simulink model "Ae483_project"  (R2018a)
settings: Solver=ode15s  StartTime=0.0  StopTime=50  RelTol=1e-4
values from neighbouring files (symbols this model uses):
  A_10_ang = [-1.3336 -0.5124 0.1399 ... (first row only)    [Ae483Project.m]
  A_10_ang_ob = bsxfun(@times, A_10_ang, [1.02; 1.04; 1.06])    [Ae483Project.m]
  A_10_full = [-0.006289	0.032720	1.318244	-32.063538	0.001827	-0.977238	0.000000	0.000733 ... (first row only)    [Ae483Project.m]
  A_80_ang = [-1.4979 -0.2372 0.4009 ... (first row only)    [Ae483Project.m]
  A_80_ang_ob = bsxfun(@times, A_80_ang, [1.02; 1.04; 1.06])    [Ae483Project.m]
  A_80_full = [-0.107611	0.120068	11.216902	-32.054340	0.007203	-0.521417	0.000000	-0.035677 ... (first row only)    [Ae483Project.m]
  B_10_ang = [-0.1712 16.8793 3.8113 ... (first row only)    [Ae483Project.m]
  B_10_ang_ob = bsxfun(@times, B_10_ang, [1.02; 1.04; 1.06])    [Ae483Project.m]
  B_10_full = [32.104822	29.961036	0.359934	0.000000 ... (first row only)    [Ae483Project.m]
  B_80_ang = [3.4190 17.0171 5.3246 ... (first row only)    [Ae483Project.m]
  B_80_ang_ob = bsxfun(@times, B_80_ang, [1.02; 1.04; 1.06])    [Ae483Project.m]
  B_80_full = [17.121858	64.081477	0.195110	0.000000 ... (first row only)    [Ae483Project.m]
  K_10 = B_10_ang^-1*(A_10_ang-A_d_ang)*C_ang^-1    [Ae483Project.m]
  K_80 = B_80_ang^-1*(A_80_ang-A_d_ang)*C_ang^-1    [Ae483Project.m]
  Ke_ang_10 = double(sym([ke1_ang_10; ke2_ang_10; ke3_ang_10]))    [Ae483Project.m]
  Ke_ang_80 = double(sym([ke1_ang_80; ke2_ang_80; ke3_ang_80]))    [Ae483Project.m]
  L_bv_10 = [cos(theta_10)*cos(psi_10), cos(theta_10)*sin(psi_10), -sin(theta_10) ... (first row only)    [Ae483Project.m]
  L_vb_10 = L_bv_10'    [Ae483Project.m]
undefined symbols (not defined in the file or in its folder): K_lqr_10, K_lqr_10_full, K_lqr_80, K_lqr_80_full
(part 2 of 2)

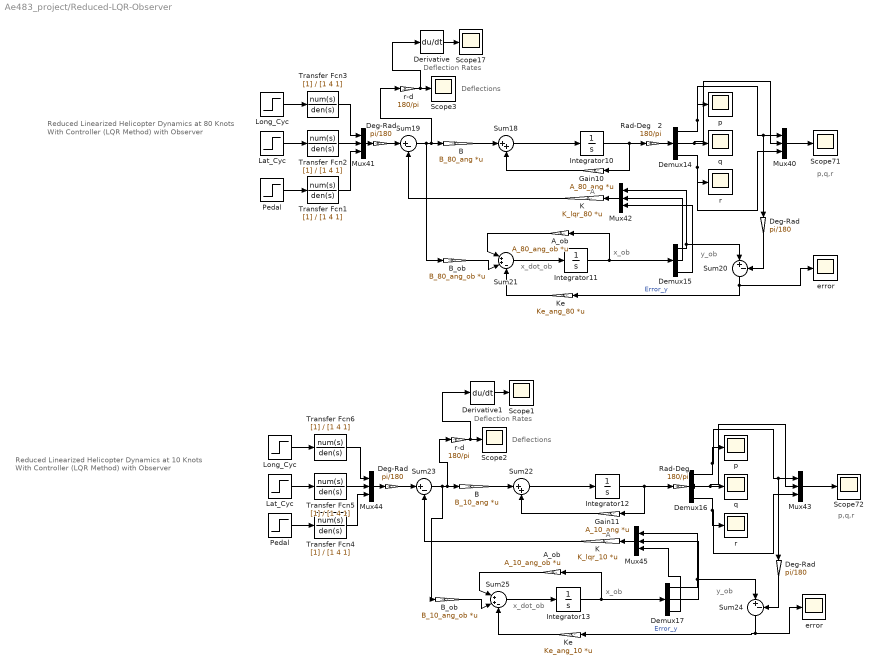
== system Ae483_project/Reduced-LQR-Observer ==
  note: A
  note: p,q,r
  note: x_ob
  note: x_dot_ob
  note: y_ob
  note: Reduced Linearized Helicopter
      | Dynamics at 80 Knots
      | With Controller
      | (LQR Method) with Observer
  note: x_dot_ob
  note: y_ob
  note: x_ob
  note: p,q,r
  note: A
  note: Reduced Linearized Helicopter
      | Dynamics at 10 Knots
      | With Controller
      | (LQR Method) with Observer
  note: Deflections
  note: Deflection Rates
  note: Deflections
  note: Deflection Rates
  "            K  " : Gain  Gain=K_lqr_10  Multiplication=Matrix(K*u)
  "           K" : Gain  Gain=K_lqr_80  Multiplication=Matrix(K*u)
  "   B    " : Gain  Gain=B_10_ang  Multiplication=Matrix(K*u)
  "   B      " : Gain  Gain=B_80_ang  Multiplication=Matrix(K*u)
    Deg-Rad {,,,} (4 alike) : Gain  Gain=pi/180
  "  Rad-Deg      " : Gain  Gain=180/pi
  "  Rad-Deg   2" : Gain  Gain=180/pi
  "  r " : Scope
  "  r   " : Scope
  " p" : Scope
  " p     " : Scope
  " q " : Scope
  " q     " : Scope
  " r-d   " : Gain  Gain=180/pi
  " r-d    " : Gain  Gain=180/pi
  A_ob : Gain  Gain=A_80_ang_ob  Multiplication=Matrix(K*u)
  "A_ob  " : Gain  Gain=A_10_ang_ob  Multiplication=Matrix(K*u)
  B_ob : Gain  Gain=B_80_ang_ob  Multiplication=Matrix(K*u)
  "B_ob " : Gain  Gain=B_10_ang_ob  Multiplication=Matrix(K*u)
  Demux{14..17} (4 alike) : Demux  Outputs=3
  Derivative : Derivative
  Derivative1 : Derivative
  Gain10 : Gain  Gain=A_80_ang  Multiplication=Matrix(K*u)
  Gain11 : Gain  Gain=A_10_ang  Multiplication=Matrix(K*u)
  Integrator{10..13} (4 alike) : Integrator
  Ke : Gain  Description=K  Gain=Ke_ang_80  Multiplication=Matrix(K*u)
  "Ke  " : Gain  Description=K  Gain=Ke_ang_10  Multiplication=Matrix(K*u)
  "Lat_Cyc " : Step  SampleTime=0
  "Lat_Cyc   " : Step  SampleTime=0
  "Long_Cyc " : Step  SampleTime=0
  "Long_Cyc   " : Step  SampleTime=0
  Mux{40..45} (6 alike) : Mux  Inputs=3
  Pedal : Step  SampleTime=0
  "Pedal   " : Step  SampleTime=0
  Scope{1..3,17,71..72} (6 alike) : Scope
  Sum18 : Sum  Inputs=|++
  Sum{19..20,23..24} (4 alike) : Sum  Inputs=|+-
  Sum21 : Sum  Inputs=|++-
  Sum22 : Sum  Inputs=|++
  Sum25 : Sum  Inputs=|++-
  Transfer Fcn{1..6} (6 alike) : TransferFcn  Denominator=[1 4 1]
  error : Scope
  "error   " : Scope
  wires:
  "A_ob  "/1 -> Sum25/1
  "           K"/1 -> Sum19/2
  Integrator12/1 -> Gain11/1, "  Rad-Deg      "/1
  Sum24/1 -> "Ke  "/1, "error   "/1  "Error_y"
  Ke/1 -> Sum21/3
  Demux17/1 -> Mux45/1, Sum24/1
  Mux41/1 -> "  Deg-Rad "/1
  Demux14/1 -> Mux40/1, "  Deg-Rad "/1, " p"/1
  "  Deg-Rad "/1 -> Sum24/2
  Sum22/1 -> Integrator12/1
  Demux15/3 -> Mux42/3
  Integrator13/1 -> Demux17/1, "A_ob  "/1
  Demux16/2 -> Mux43/2, " q     "/1
  Demux17/3 -> Mux45/3
  Demux14/2 -> Mux40/2, " q "/1
  Sum25/1 -> Integrator13/1
  "   B      "/1 -> Sum18/1
  "Long_Cyc   "/1 -> Transfer Fcn6/1
  "Pedal   "/1 -> Transfer Fcn4/1
  Mux43/1 -> Scope72/1
  Mux40/1 -> Scope71/1
  Sum18/1 -> Integrator10/1
  "  Rad-Deg      "/1 -> Demux16/1
  Demux16/3 -> Mux43/3, "  r   "/1
  "  Deg-Rad "/1 -> Sum20/2
  Mux45/1 -> "            K  "/1
  Demux16/1 -> Mux43/1, "  Deg-Rad "/1, " p     "/1
  Demux17/2 -> Mux45/2
  Sum23/1 -> "B_ob "/1, " r-d   "/1, "   B    "/1
  Gain10/1 -> Sum18/2
  "   B    "/1 -> Sum22/1
  Demux14/3 -> Mux40/3, "  r "/1
  "  Deg-Rad "/1 -> Sum23/1
  "B_ob "/1 -> Sum25/2
  "  Deg-Rad "/1 -> Sum19/1
  "Ke  "/1 -> Sum25/3
  Integrator10/1 -> Gain10/1, "  Rad-Deg   2"/1
  "            K  "/1 -> Sum23/2
  Mux44/1 -> "  Deg-Rad "/1
  Gain11/1 -> Sum22/2
  Integrator11/1 -> Demux15/1, A_ob/1
  A_ob/1 -> Sum21/1
  Sum21/1 -> Integrator11/1
  "  Rad-Deg   2"/1 -> Demux14/1
  Demux15/2 -> Mux42/2
  B_ob/1 -> Sum21/2
  Sum20/1 -> Ke/1, error/1  "Error_y"
  Mux42/1 -> "           K"/1
  Demux15/1 -> Mux42/1, Sum20/1
  Transfer Fcn4/1 -> Mux44/3
  Transfer Fcn6/1 -> Mux44/1
  "Lat_Cyc   "/1 -> Transfer Fcn5/1
  Transfer Fcn5/1 -> Mux44/2
  Transfer Fcn2/1 -> Mux41/2
  "Lat_Cyc "/1 -> Transfer Fcn2/1
  Transfer Fcn3/1 -> Mux41/1
  Transfer Fcn1/1 -> Mux41/3
  Pedal/1 -> Transfer Fcn1/1
  "Long_Cyc "/1 -> Transfer Fcn3/1
  Derivative1/1 -> Scope1/1
  " r-d   "/1 -> Derivative1/1, Scope2/1
  " r-d    "/1 -> Derivative/1, Scope3/1
  Sum19/1 -> B_ob/1, " r-d    "/1, "   B      "/1
  Derivative/1 -> Scope17/1

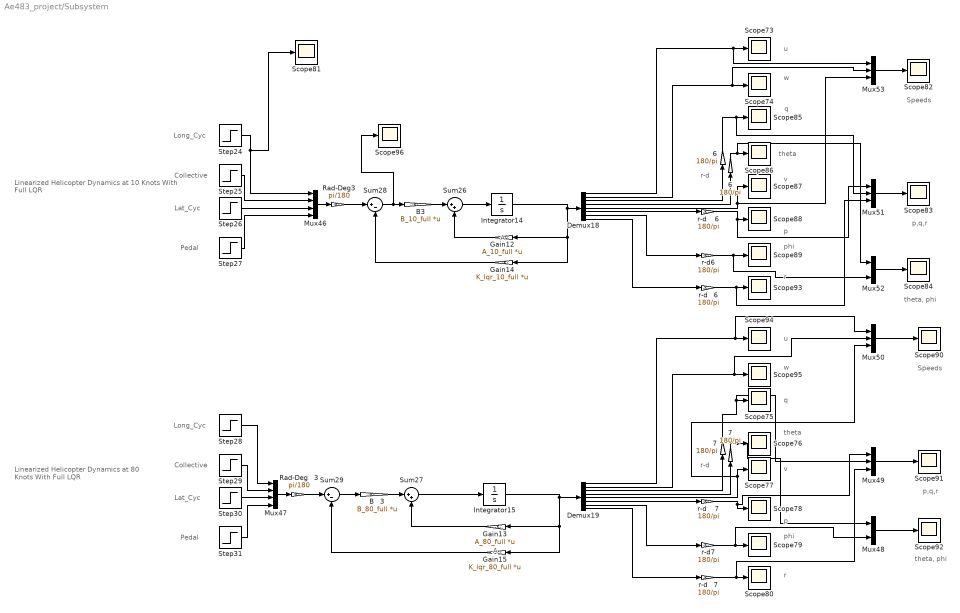
== system Ae483_project/Subsystem ==
  note: Linearized Helicopter
      | Dynamics at 10 Knots
      | With Full LQR
  note: q
  note: Speeds
  note: A
  note: r
  note: Linearized Helicopter
      | Dynamics at 80 Knots
      | With Full LQR
  note: w
  note: r-d
  note: phi
  note: Long_Cyc
  note: theta
  note: Speeds
  note: Pedal
  note: Long_Cyc
  note: p,q,r
  note: Pedal
  note: theta
  note: p
  note: u
  note: r
  note: q
  note: v
  note: Lat_Cyc
  note: u
  note: w
  note: phi
  note: theta, phi
  note: Collective
  note: p
  note: Collective
  note: Lat_Cyc
  note: p,q,r
  note: v
  note: A
  note: theta, phi
  note: r-d
  "    6" : Gain  Gain=180/pi
  "    7" : Gain  Gain=180/pi
  " 6" : Gain  Gain=180/pi
  " 7" : Gain  Gain=180/pi
  " r-d   6" : Gain  Gain=180/pi
  " r-d   7" : Gain  Gain=180/pi
  " r-d6" : Gain  Gain=180/pi
  " r-d7" : Gain  Gain=180/pi
  B   3 : Gain  Gain=B_80_full  Multiplication=Matrix(K*u)
  B3 : Gain  Gain=B_10_full  Multiplication=Matrix(K*u)
  Demux18 : Demux  Outputs=8
  Demux19 : Demux  Outputs=8
  Gain12 : Gain  Gain=A_10_full  Multiplication=Matrix(K*u)
  Gain13 : Gain  Gain=A_80_full  Multiplication=Matrix(K*u)
  Gain14 : Gain  Gain=K_lqr_10_full  Multiplication=Matrix(K*u)
  Gain15 : Gain  Gain=K_lqr_80_full  Multiplication=Matrix(K*u)
  Integrator14 : Integrator
  Integrator15 : Integrator
  Mux46 : Mux
  Mux47 : Mux
  Mux48 : Mux  Inputs=2
  Mux{49..51,53} (4 alike) : Mux  Inputs=3
  Mux52 : Mux  Inputs=2
  Rad-Deg   3 : Gain  Gain=pi/180
  Rad-Deg3 : Gain  Gain=pi/180
  Scope{73..96} (24 alike) : Scope
  Step{24..27} (4 alike) : Step  After=10  SampleTime=0
  Step{28..31} (4 alike) : Step  SampleTime=0
  Sum26 : Sum  Inputs=|++
  Sum27 : Sum  Inputs=|++
  Sum28 : Sum  Inputs=|+-
  Sum29 : Sum  Inputs=|+-
  r-d    6 : Gain  Gain=180/pi
  r-d    7 : Gain  Gain=180/pi
  wires:
  Demux19/5 -> Mux50/3, Scope77/1
  r-d    6/1 -> Mux51/1, Scope88/1
  Demux18/8 -> " r-d   6"/1
  Demux19/7 -> " r-d7"/1
  r-d    7/1 -> Mux49/1, Scope78/1
  Demux19/3 -> " 7"/1
  Integrator15/1 -> Demux19/1, Gain15/1, Gain13/1
  Step24/1 -> Scope81/1, Mux46/1
  Step30/1 -> Mux47/3
  Mux46/1 -> Rad-Deg3/1
  Demux18/5 -> Mux53/3, Scope87/1
  Demux18/4 -> "    6"/1
  Sum26/1 -> Integrator14/1
  Gain14/1 -> Sum28/2
  Sum28/1 -> Scope96/1, B3/1
  Step26/1 -> Mux46/3
  " 7"/1 -> Mux49/2, Scope75/1
  " 6"/1 -> Mux51/2, Scope85/1
  "    7"/1 -> Mux48/1, Scope76/1
  Demux18/1 -> Mux53/1, Scope73/1
  Mux50/1 -> Scope90/1
  Demux19/4 -> "    7"/1
  " r-d   7"/1 -> Mux49/3, Scope80/1
  " r-d   6"/1 -> Mux51/3, Scope93/1
  " r-d6"/1 -> Mux52/2, Scope89/1
  Step25/1 -> Mux46/2
  Step27/1 -> Mux46/4
  " r-d7"/1 -> Mux48/2, Scope79/1
  Sum27/1 -> Integrator15/1
  Mux49/1 -> Scope91/1
  Demux18/2 -> Mux53/2, Scope74/1
  Mux51/1 -> Scope83/1
  Integrator14/1 -> Demux18/1, Gain14/1, Gain12/1
  Demux19/2 -> Mux50/2, Scope95/1
  Gain12/1 -> Sum26/2
  Mux52/1 -> Scope84/1
  B3/1 -> Sum26/1
  Demux19/6 -> r-d    7/1
  Step29/1 -> Mux47/2
  Demux18/7 -> " r-d6"/1
  B   3/1 -> Sum27/1
  "    6"/1 -> Mux52/1, Scope86/1
  Mux48/1 -> Scope92/1
  Demux19/1 -> Mux50/1, Scope94/1
  Demux18/3 -> " 6"/1
  Demux19/8 -> " r-d   7"/1
  Rad-Deg3/1 -> Sum28/1
  Step31/1 -> Mux47/4
  Demux18/6 -> r-d    6/1
  Gain15/1 -> Sum29/2
  Mux53/1 -> Scope82/1
  Rad-Deg   3/1 -> Sum29/1
  Sum29/1 -> B   3/1
  Gain13/1 -> Sum27/2
  Mux47/1 -> Rad-Deg   3/1
  Step28/1 -> Mux47/1

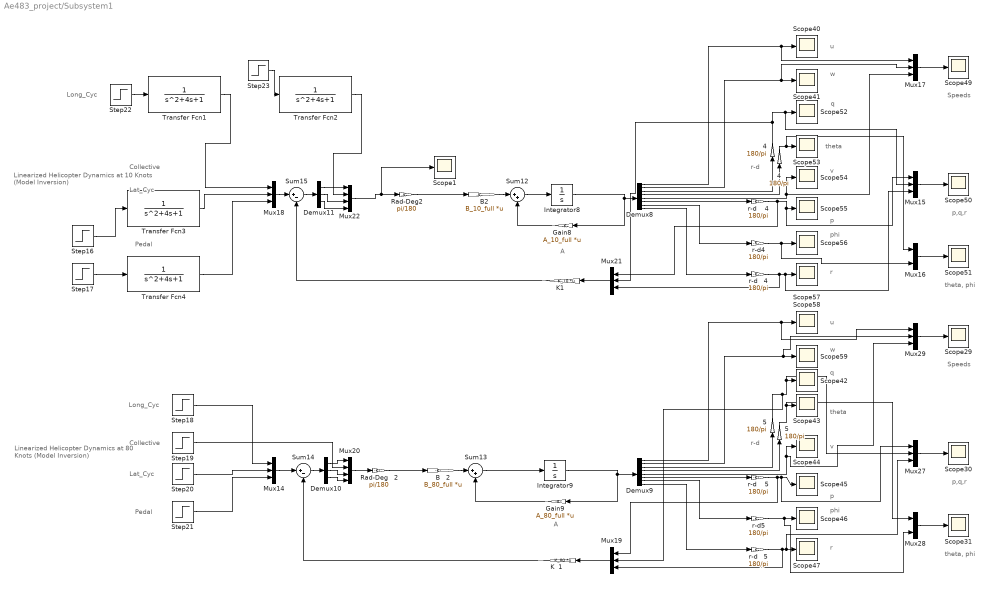
== system Ae483_project/Subsystem1 ==
  note: A
  note: v
  note: p,q,r
  note: phi
  note: Speeds
  note: Pedal
  note: u
  note: Collective
  note: Lat_Cyc
  note: r-d
  note: Collective
  note: Long_Cyc
  note: q
  note: theta
  note: w
  note: r
  note: theta
  note: u
  note: w
  note: Linearized Helicopter
      | Dynamics at 80 Knots
      | (Model Inversion)
  note: q
  note: Pedal
  note: Lat_Cyc
  note: r-d
  note: theta, phi
  note: Long_Cyc
  note: r
  note: phi
  note: p
  note: Linearized Helicopter
      | Dynamics at 10 Knots
      | (Model Inversion)
  note: A
  note: v
  note: p
  note: p,q,r
  note: Speeds
  note: theta, phi
  "         K  1" : Gain  Gain=K_80  Multiplication=Matrix(K*u)
  "    4" : Gain  Gain=180/pi
  "    5" : Gain  Gain=180/pi
  "    K1" : Gain  Gain=K_10  Multiplication=Matrix(K*u)
  " 4" : Gain  Gain=180/pi
  " 5" : Gain  Gain=180/pi
  " r-d   4" : Gain  Gain=180/pi
  " r-d   5" : Gain  Gain=180/pi
  " r-d4" : Gain  Gain=180/pi
  " r-d5" : Gain  Gain=180/pi
  B   2 : Gain  Gain=B_80_full  Multiplication=Matrix(K*u)
  B2 : Gain  Gain=B_10_full  Multiplication=Matrix(K*u)
  Demux10 : Demux  Outputs=3
  Demux11 : Demux  Outputs=3
  Demux8 : Demux  Outputs=8
  Demux9 : Demux  Outputs=8
  Gain8 : Gain  Gain=A_10_full  Multiplication=Matrix(K*u)
  Gain9 : Gain  Gain=A_80_full  Multiplication=Matrix(K*u)
  Integrator8 : Integrator
  Integrator9 : Integrator
  Mux{14..15,17..19,21,27,29} (8 alike) : Mux  Inputs=3
  Mux16 : Mux  Inputs=2
  Mux20 : Mux
  Mux22 : Mux
  Mux28 : Mux  Inputs=2
  Rad-Deg   2 : Gain  Gain=pi/180
  Rad-Deg2 : Gain  Gain=pi/180
  Scope{1,29..31,40..47,49..59} (23 alike) : Scope
  Step16 : Step  After=5  SampleTime=0
  Step17 : Step  After=5  SampleTime=0
  Step{18..21} (4 alike) : Step  SampleTime=0
  Step22 : Step  After=5  SampleTime=0
  Step23 : Step  After=10  SampleTime=0
  Sum12 : Sum  Inputs=|++
  Sum13 : Sum  Inputs=|++
  Sum14 : Sum  Inputs=|+-
  Sum15 : Sum  Inputs=|+-
  Transfer Fcn{1..4} (4 alike) : TransferFcn  Denominator=[1 4 1]
  r-d    4 : Gain  Gain=180/pi
  r-d    5 : Gain  Gain=180/pi
  wires:
  Demux11/2 -> Mux22/3
  "         K  1"/1 -> Sum14/2
  Demux8/4 -> "    4"/1
  Gain9/1 -> Sum13/2
  " 5"/1 -> Mux19/2, Mux27/2, Scope42/1
  Demux10/2 -> Mux20/3
  Mux20/1 -> Rad-Deg   2/1
  r-d    4/1 -> Mux21/1, Mux15/1, Scope55/1
  r-d    5/1 -> Mux19/1, Mux27/1, Scope45/1
  Demux9/4 -> "    5"/1
  B2/1 -> Sum12/1
  Demux8/3 -> " 4"/1
  Mux21/1 -> "    K1"/1
  Gain8/1 -> Sum12/2
  Demux8/2 -> Mux17/2, Scope41/1
  Mux14/1 -> Sum14/1
  Mux22/1 -> Scope1/1, Rad-Deg2/1
  Demux9/8 -> " r-d   5"/1
  " r-d4"/1 -> Mux16/2, Scope56/1
  Step22/1 -> Transfer Fcn1/1
  "    5"/1 -> Mux28/1, Scope43/1
  Mux15/1 -> Scope50/1
  Integrator8/1 -> Demux8/1, Gain8/1
  Step18/1 -> Mux14/1
  Demux8/1 -> Mux17/1, Scope40/1
  " r-d   4"/1 -> Mux21/3, Mux15/3, Scope57/1
  Step20/1 -> Mux14/2
  "    K1"/1 -> Sum15/2
  Sum13/1 -> Integrator9/1
  Demux8/6 -> r-d    4/1
  Demux9/7 -> " r-d5"/1
  Mux16/1 -> Scope51/1
  Demux9/3 -> " 5"/1
  Sum15/1 -> Demux11/1
  Demux9/5 -> Mux29/3, Scope44/1
  Step19/1 -> Mux20/2
  Demux8/8 -> " r-d   4"/1
  " r-d5"/1 -> Mux28/2, Scope46/1
  Integrator9/1 -> Demux9/1, Gain9/1
  Step17/1 -> Transfer Fcn4/1
  " r-d   5"/1 -> Mux19/3, Mux27/3, Scope47/1
  Demux9/6 -> r-d    5/1
  Rad-Deg   2/1 -> B   2/1
  Demux10/3 -> Mux20/4
  " 4"/1 -> Mux15/2, Scope52/1, Mux21/2
  Demux9/2 -> Mux29/2, Scope59/1
  Sum12/1 -> Integrator8/1
  "    4"/1 -> Mux16/1, Scope53/1
  Mux18/1 -> Sum15/1
  Mux17/1 -> Scope49/1
  Demux8/5 -> Mux17/3, Scope54/1
  Demux8/7 -> " r-d4"/1
  B   2/1 -> Sum13/1
  Step21/1 -> Mux14/3
  Mux19/1 -> "         K  1"/1
  Step16/1 -> Transfer Fcn3/1
  Sum14/1 -> Demux10/1
  Demux10/1 -> Mux20/1
  Mux28/1 -> Scope31/1
  Mux29/1 -> Scope29/1
  Demux11/1 -> Mux22/1
  Mux27/1 -> Scope30/1
  Demux11/3 -> Mux22/4
  Demux9/1 -> Mux29/1, Scope58/1
  Step23/1 -> Transfer Fcn2/1
  Rad-Deg2/1 -> B2/1
  Transfer Fcn1/1 -> Mux18/1
  Transfer Fcn2/1 -> Mux22/2
  Transfer Fcn3/1 -> Mux18/2
  Transfer Fcn4/1 -> Mux18/3

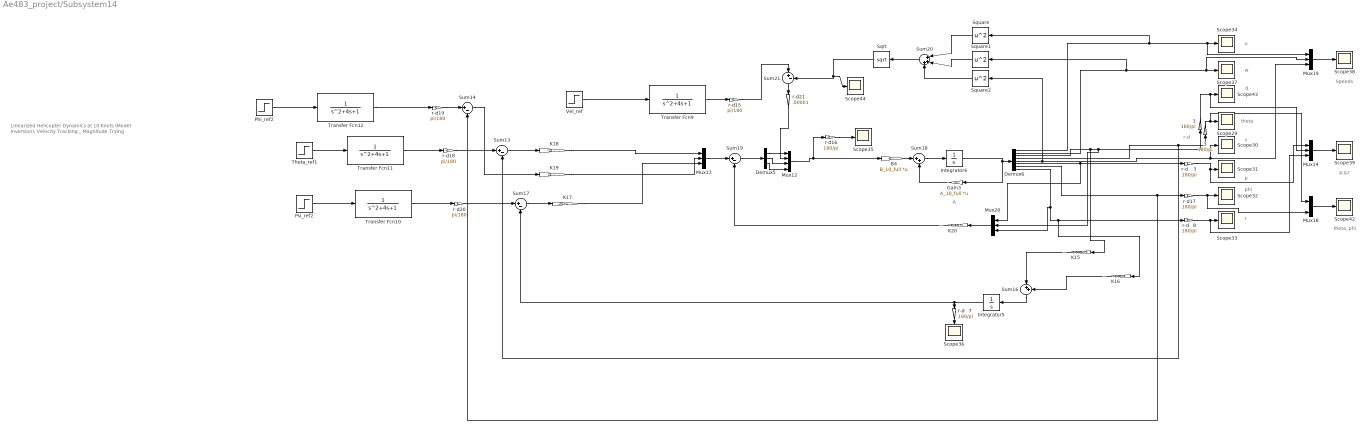
== system Ae483_project/Subsystem14 ==
  note: theta
  note: A
  note: Speeds
  note: r
  note: r-d
  note: p,q,r
  note: phi
  note: q
  note: w
  note: v
  note: p
  note: theta, phi
  note: u
  note: Linearized Helicopter
      | Dynamics at 10 Knots
      | (Model Inversion), Velocity Tracking _ Magnitude Trying
  "    3" : Gain  Gain=180/pi
  "    K15" : Gain  Gain=0.000629
  "    K16" : Gain  Gain=1.0024
  "    K17" : Gain  Gain=-25  Multiplication=Matrix(K*u)
  "    K18" : Gain  Gain=-15
  "    K19" : Gain  Gain=15
  "    K20" : Gain  Gain=K_10  Multiplication=Matrix(K*u)
  " 3" : Gain  Gain=180/pi
  " r-d   7" : Gain  Gain=180/pi
  " r-d   8" : Gain  Gain=180/pi
   r-d{15,18..20} (4 alike) : Gain  Gain=pi/180
  " r-d16" : Gain  Gain=180/pi
  " r-d17" : Gain  Gain=180/pi
  " r-d21" : Gain  Gain=.00001
  B4 : Gain  Gain=B_10_full  Multiplication=Matrix(K*u)
  Demux5 : Demux  Outputs=3
  Demux6 : Demux  Outputs=8
  Gain3 : Gain  Gain=A_10_full  Multiplication=Matrix(K*u)
  Integrator5 : Integrator
  Integrator6 : Integrator
  Mux12 : Mux
  Mux{13..14,19..20} (4 alike) : Mux  Inputs=3
  Mux18 : Mux  Inputs=2
  Phi_ref2 : Step  After=8  SampleTime=0
  Psi_ref2 : Step  After=15  SampleTime=0
  Scope{29..39,42..44} (14 alike) : Scope
  Sqrt : Sqrt  SaturateOnIntegerOverflow=on
  Square : Math  Operator=square  SaturateOnIntegerOverflow=on
  Square1 : Math  Operator=square  SaturateOnIntegerOverflow=on
  Square2 : Math  Operator=square  SaturateOnIntegerOverflow=on
  Sum{13..14,17,19,21} (5 alike) : Sum  Inputs=|+-
  Sum16 : Sum  Inputs=|++
  Sum18 : Sum  Inputs=|++
  Sum20 : Sum  Inputs=|+++
  Theta_ref1 : Step  After=5  SampleTime=0
  Transfer Fcn{9..12} (4 alike) : TransferFcn  Denominator=[1 4 1]
  Vel_ref : Step  After=15  SampleTime=0
  r-d    3 : Gain  Gain=180/pi
  wires:
  "    K18"/1 -> Mux13/1
  Sum21/1 -> " r-d21"/1
  Demux6/2 -> Square1/1, Mux19/2, Scope37/1
  Demux6/7 -> Sum14/2, " r-d17"/1
  Sum18/1 -> Integrator6/1
  Transfer Fcn10/1 -> " r-d20"/1
  Mux14/1 -> Scope39/1
  Mux19/1 -> Scope38/1
  Integrator6/1 -> Demux6/1, Gain3/1
  Sum20/1 -> Sqrt/1
  r-d    3/1 -> Mux14/1, Scope31/1
  Mux12/1 -> B4/1, " r-d16"/1
  Demux6/8 -> Mux20/3, "    K16"/1, " r-d   8"/1
  Sum17/1 -> "    K17"/1
  " r-d19"/1 -> Sum14/1
  Demux6/1 -> Square/1, Scope34/1, Mux19/1
  Mux18/1 -> Scope42/1
  Psi_ref2/1 -> Transfer Fcn10/1
  B4/1 -> Sum18/1
  Sum19/1 -> Demux5/1
  Demux5/1 -> Mux12/1
  "    K16"/1 -> Sum16/2
  Demux6/5 -> Square2/1, Mux19/3, Scope30/1
  Demux6/6 -> Mux20/1, r-d    3/1
  Demux6/3 -> "    K15"/1, Mux20/2, " 3"/1
  Integrator5/1 -> " r-d   7"/1, Sum17/2
  " 3"/1 -> Mux14/2, Scope43/1
  Square1/1 -> Sum20/2
  Mux13/1 -> Sum19/1
  Transfer Fcn12/1 -> " r-d19"/1
  "    K17"/1 -> Mux13/3
  Demux5/2 -> Mux12/3
  "    3"/1 -> Mux18/1, Scope29/1
  " r-d   8"/1 -> Mux14/3, Scope33/1
  "    K19"/1 -> Mux13/2
  Transfer Fcn9/1 -> " r-d15"/1
  Phi_ref2/1 -> Transfer Fcn12/1
  Square2/1 -> Sum20/3
  " r-d15"/1 -> Sum21/1
  " r-d17"/1 -> Mux18/2, Scope32/1
  " r-d21"/1 -> Mux12/2
  Gain3/1 -> Sum18/2
  Sum16/1 -> Integrator5/1
  "    K20"/1 -> Sum19/2
  " r-d   7"/1 -> Scope36/1
  Transfer Fcn11/1 -> " r-d18"/1
  Theta_ref1/1 -> Transfer Fcn11/1
  Sum14/1 -> "    K19"/1
  Sqrt/1 -> Scope44/1, Sum21/2
  " r-d18"/1 -> Sum13/1
  Square/1 -> Sum20/1
  " r-d20"/1 -> Sum17/1
  "    K15"/1 -> Sum16/1
  Demux5/3 -> Mux12/4
  Demux6/4 -> Sum13/2, "    3"/1
  " r-d16"/1 -> Scope35/1
  Mux20/1 -> "    K20"/1
  Vel_ref/1 -> Transfer Fcn9/1
  Sum13/1 -> "    K18"/1

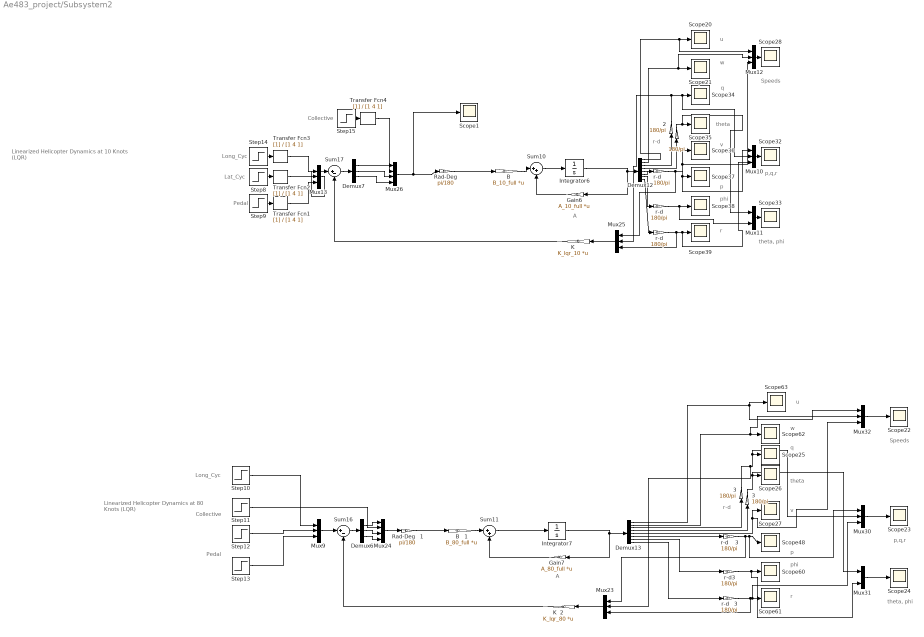
== system Ae483_project/Subsystem2 ==
  note: Linearized Helicopter
      | Dynamics at 10 Knots
      | (LQR)
  note: Linearized Helicopter
      | Dynamics at 80 Knots
      | (LQR)
  note: A
  note: p,q,r
  note: phi
  note: Speeds
  note: Pedal
  note: u
  note: Lat_Cyc
  note: r-d
  note: Collective
  note: Long_Cyc
  note: q
  note: theta
  note: w
  note: r
  note: Pedal
  note: theta, phi
  note: p
  note: v
  note: Speeds
  note: p,q,r
  note: p
  note: A
  note: r
  note: phi
  note: Long_Cyc
  note: r-d
  note: q
  note: theta
  note: w
  note: theta, phi
  note: Collective
  note: v
  note: u
  "       " : Gain  Gain=180/pi
  "         K  2" : Gain  Gain=K_lqr_80  Multiplication=Matrix(K*u)
  "    3" : Gain  Gain=180/pi
  "    K  " : Gain  Gain=K_lqr_10  Multiplication=Matrix(K*u)
  " 2" : Gain  Gain=180/pi
  " 3" : Gain  Gain=180/pi
  " r-d " : Gain  Gain=180/pi
  " r-d   " : Gain  Gain=180/pi
  " r-d   3" : Gain  Gain=180/pi
  " r-d3" : Gain  Gain=180/pi
  "B  " : Gain  Gain=B_10_full  Multiplication=Matrix(K*u)
  B   1 : Gain  Gain=B_80_full  Multiplication=Matrix(K*u)
  Demux12 : Demux  Outputs=8
  Demux13 : Demux  Outputs=8
  Demux6 : Demux  Outputs=3
  Demux7 : Demux  Outputs=3
  Gain6 : Gain  Gain=A_10_full  Multiplication=Matrix(K*u)
  Gain7 : Gain  Gain=A_80_full  Multiplication=Matrix(K*u)
  Integrator6 : Integrator
  Integrator7 : Integrator
  Mux{9..10,12..13,23,25,30,32} (8 alike) : Mux  Inputs=3
  Mux11 : Mux  Inputs=2
  Mux24 : Mux
  Mux26 : Mux
  Mux31 : Mux  Inputs=2
  "Rad-Deg  " : Gain  Gain=pi/180
  Rad-Deg   1 : Gain  Gain=pi/180
  Scope{1,20..28,32..39,48,60..63} (23 alike) : Scope
  Step{10..13} (4 alike) : Step  SampleTime=0
  Step14 : Step  After=0  SampleTime=0
  Step15 : Step  After=10  SampleTime=0
  Step8 : Step  After=0  SampleTime=0
  Step9 : Step  After=0  SampleTime=0
  Sum10 : Sum  Inputs=|++
  Sum11 : Sum  Inputs=|++
  Sum16 : Sum  Inputs=|+-
  Sum17 : Sum  Inputs=|+-
  Transfer Fcn{1..4} (4 alike) : TransferFcn  Denominator=[1 4 1]
  "r-d      " : Gain  Gain=180/pi
  r-d    3 : Gain  Gain=180/pi
  wires:
  Mux23/1 -> "         K  2"/1
  Mux13/1 -> Sum17/1
  " r-d   3"/1 -> Mux23/3, Mux30/3, Scope61/1
  Demux13/6 -> r-d    3/1
  " r-d3"/1 -> Mux31/2, Scope60/1
  Mux26/1 -> Scope1/1, "Rad-Deg  "/1
  Step13/1 -> Mux9/3
  " 3"/1 -> Mux23/2, Mux30/2, Scope25/1
  Demux12/6 -> "r-d      "/1
  Demux6/1 -> Mux24/1
  Demux12/7 -> " r-d   "/1
  Demux13/7 -> " r-d3"/1
  Mux31/1 -> Scope24/1
  Mux24/1 -> Rad-Deg   1/1
  Demux6/3 -> Mux24/4
  Demux12/3 -> " 2"/1
  Mux11/1 -> Scope33/1
  Demux13/3 -> " 3"/1
  Demux13/1 -> Scope63/1, Mux32/1
  Gain6/1 -> Sum10/2
  Mux9/1 -> Sum16/1
  " r-d "/1 -> Scope39/1, Mux10/3, Mux25/3
  " 2"/1 -> Mux25/2, Scope34/1, Mux10/2
  Integrator6/1 -> Gain6/1, Demux12/1
  Demux12/8 -> " r-d "/1
  "Rad-Deg  "/1 -> "B  "/1
  "B  "/1 -> Sum10/1
  Step10/1 -> Mux9/1
  "r-d      "/1 -> Scope37/1, Mux10/1, Mux25/1
  Step11/1 -> Mux24/2
  Integrator7/1 -> Demux13/1, Gain7/1
  Demux13/4 -> "    3"/1
  Mux32/1 -> Scope22/1
  Demux12/4 -> "       "/1
  " r-d   "/1 -> Scope38/1, Mux11/2
  Demux12/5 -> Scope36/1, Mux12/3
  Demux13/5 -> Mux32/3, Scope27/1
  r-d    3/1 -> Mux23/1, Mux30/1, Scope48/1
  Sum11/1 -> Integrator7/1
  Step12/1 -> Mux9/2
  Mux25/1 -> "    K  "/1
  Demux13/2 -> Mux32/2, Scope62/1
  Mux30/1 -> Scope23/1
  "    3"/1 -> Mux31/1, Scope26/1
  Demux12/2 -> Scope21/1, Mux12/2
  Mux10/1 -> Scope32/1
  "       "/1 -> Scope35/1, Mux11/1
  "         K  2"/1 -> Sum16/2
  Demux13/8 -> " r-d   3"/1
  Demux7/2 -> Mux26/3
  Sum16/1 -> Demux6/1
  Gain7/1 -> Sum11/2
  Mux12/1 -> Scope28/1
  Sum17/1 -> Demux7/1
  Sum10/1 -> Integrator6/1
  Rad-Deg   1/1 -> B   1/1
  Demux7/3 -> Mux26/4
  Demux7/1 -> Mux26/1
  "    K  "/1 -> Sum17/2
  B   1/1 -> Sum11/1
  Demux12/1 -> Scope20/1, Mux12/1
  Demux6/2 -> Mux24/3
  Step15/1 -> Transfer Fcn4/1
  Step14/1 -> Transfer Fcn3/1
  Step8/1 -> Transfer Fcn2/1
  Step9/1 -> Transfer Fcn1/1
  Transfer Fcn1/1 -> Mux13/3
  Transfer Fcn2/1 -> Mux13/2
  Transfer Fcn3/1 -> Mux13/1
  Transfer Fcn4/1 -> Mux26/2

== system Ae483_project/Subsystem7 ==
  note: A
  note: p,q,r
  note: Reduced Linearized Helicopter
      | Dynamics at 10 Knots
      | With Controller
      | (LQR Method) Heading, Tracking Control
  note: p,q,r
  note: Reduced Linearized Helicopter
      | Dynamics at 80 Knots
      | With Controller
      | (LQR Method) Heading, Tracking Control
  note: A
  "     K 1" : Gain  Gain=K_lqr_10  Multiplication=Matrix(K*u)
  "     K 2" : Gain  Gain=[0; 0; -10000]  Multiplication=Matrix(K*u)
  "     K 5" : Gain  Gain=K_lqr_80  Multiplication=Matrix(K*u)
  "     K 6" : Gain  Gain=[0; 0; -10000]  Multiplication=Matrix(K*u)
    Rad-Deg   {4..7} (4 alike) : Gain  Gain=180/pi
  B      1 : Gain  Gain=B_10_ang  Multiplication=Matrix(K*u)
  B      2 : Gain  Gain=B_80_ang  Multiplication=Matrix(K*u)
  Demux1 : Demux  Outputs=3
  Demux20 : Demux  Outputs=3
  Gain1 : Gain  Gain=A_80_ang  Multiplication=Matrix(K*u)
  Gain16 : Gain  Gain=A_10_ang  Multiplication=Matrix(K*u)
  Integrator1 : Integrator
  Integrator16 : Integrator
  Mux55 : Mux  Inputs=3
  Mux6 : Mux  Inputs=3
  Rad-Deg       1 : Gain  Gain=pi/180
  Rad-Deg       2 : Gain  Gain=pi/180
  Scope{1,24..25,97..98} (5 alike) : Scope
  Sum1 : Sum  Inputs=|++
  Sum{10..11,31..32} (4 alike) : Sum  Inputs=|+-
  Sum30 : Sum  Inputs=|++
  Transfer Fcn1 : TransferFcn  Denominator=[1 4 1]
  Transfer Fcn4 : TransferFcn  Denominator=[1 4 1]
  p 1 : Scope
  p 2 : Scope
  q  1 : Scope
  q  2 : Scope
  r  1 : Scope
  r  2 : Scope
  r_ref : Step  After=5  SampleTime=0
  r_ref1 : Step  After=5  SampleTime=0
  wires:
  "     K 6"/1 -> Sum10/1
  Sum31/1 -> B      1/1, "  Rad-Deg   5"/1
  Sum10/1 -> B      2/1, "  Rad-Deg   7"/1
  Demux1/1 -> Mux6/1, p 2/1
  Transfer Fcn1/1 -> Scope1/1, Sum32/1
  Demux1/2 -> Mux6/2, q  2/1
  Demux1/3 -> Mux6/3, Sum11/2, r  2/1
  "     K 1"/1 -> Sum31/2
  "     K 2"/1 -> Sum31/1
  Sum11/1 -> Rad-Deg       1/1
  Demux20/3 -> Mux55/3, Sum32/2, r  1/1
  Gain16/1 -> Sum30/2
  Demux20/2 -> Mux55/2, q  1/1
  "  Rad-Deg   6"/1 -> Demux1/1
  Mux6/1 -> Scope24/1
  Sum1/1 -> Integrator1/1
  Integrator1/1 -> "  Rad-Deg   6"/1, "     K 5"/1, Gain1/1
  Integrator16/1 -> "  Rad-Deg   4"/1, "     K 1"/1, Gain16/1
  B      2/1 -> Sum1/1
  "     K 5"/1 -> Sum10/2
  Transfer Fcn4/1 -> Sum11/1
  r_ref1/1 -> Transfer Fcn4/1
  Demux20/1 -> Mux55/1, p 1/1
  Rad-Deg       1/1 -> "     K 6"/1
  "  Rad-Deg   7"/1 -> Scope25/1
  Gain1/1 -> Sum1/2
  "  Rad-Deg   5"/1 -> Scope98/1
  r_ref/1 -> Transfer Fcn1/1
  Rad-Deg       2/1 -> "     K 2"/1
  Mux55/1 -> Scope97/1
  Sum32/1 -> Rad-Deg       2/1
  "  Rad-Deg   4"/1 -> Demux20/1
  B      1/1 -> Sum30/1
  Sum30/1 -> Integrator16/1

== system Ae483_project/Subsystem8 ==
  note: q
  note: r-d
  note: Speeds
  note: theta, phi
  note: u
  note: w
  note: v
  note: A
  note: r
  note: theta
  note: p,q,r
  note: phi
  note: p
  note: Linearized Helicopter
      | Dynamics at 10 Knots
      | With Full LQR, Velocity, Tracking Control
  note: Linearized Helicopter
      | Dynamics at 80 Knots
      | With Full LQR, Velocity, Tracking Control
  note: theta
  note: r
  note: phi
  note: p
  note: theta, phi
  note: Speeds
  note: q
  note: r-d
  note: w
  note: A
  note: v
  note: p,q,r
  note: u
  "     K 4" : Gain  Gain=[50; 0;0;0]  Multiplication=Matrix(K*u)
  "     K 8" : Gain  Gain=[4; 0;0;0]  Multiplication=Matrix(K*u)
  "    2" : Gain  Gain=180/pi
  "    9" : Gain  Gain=180/pi
  " 2" : Gain  Gain=180/pi
  " 9" : Gain  Gain=180/pi
   r-d   {1..2,10..11} (4 alike) : Gain  Gain=180/pi
  " r-d2" : Gain  Gain=180/pi
  " r-d9" : Gain  Gain=180/pi
  B2 : Gain  Gain=B_80_full  Multiplication=Matrix(K*u)
  B5 : Gain  Gain=B_10_full  Multiplication=Matrix(K*u)
  Demux22 : Demux  Outputs=8
  Demux7 : Demux  Outputs=8
  Gain19 : Gain  Gain=A_10_full  Multiplication=Matrix(K*u)
  Gain20 : Gain  Gain=K_lqr_10_full  Multiplication=Matrix(K*u)
  Gain8 : Gain  Gain=A_80_full  Multiplication=Matrix(K*u)
  Gain9 : Gain  Gain=K_lqr_80_full  Multiplication=Matrix(K*u)
  Integrator18 : Integrator
  Integrator7 : Integrator
  Mux{1,11,54,60} (4 alike) : Mux  Inputs=3
  Mux10 : Mux  Inputs=2
  Mux59 : Mux  Inputs=2
  Scope{12..23,111..122} (24 alike) : Scope
  Sum15 : Sum  Inputs=|++
  Sum{16..17,37..38} (4 alike) : Sum  Inputs=|+-
  Sum36 : Sum  Inputs=|++
  Transfer Fcn2 : TransferFcn  Denominator=[1 4 1]
  Transfer Fcn5 : TransferFcn  Denominator=[1 4 1]
  Uref : Step  After=25  SampleTime=0
  Uref1 : Step  After=25  SampleTime=0
  r-d    2 : Gain  Gain=180/pi
  r-d    9 : Gain  Gain=180/pi
  wires:
  Integrator18/1 -> Demux22/1, Gain20/1, Gain19/1
  Mux10/1 -> Scope16/1
  Demux22/3 -> " 9"/1
  Demux7/8 -> " r-d   1"/1
  Sum16/1 -> " r-d   2"/1, B2/1
  " 2"/1 -> Mux1/2, Scope17/1
  Transfer Fcn2/1 -> Sum38/1
  Demux22/1 -> Mux60/1, Scope122/1, Sum38/2
  Demux7/1 -> Mux11/1, Scope23/1, Sum17/2
  Gain8/1 -> Sum15/2
  " 9"/1 -> Mux54/2, Scope116/1
  B5/1 -> Sum36/1
  Demux7/6 -> r-d    2/1
  Demux22/5 -> Mux60/3, Scope118/1
  " r-d   1"/1 -> Mux1/3, Scope22/1
  Demux7/5 -> Mux11/3, Scope19/1
  Sum37/1 -> " r-d   11"/1, B5/1
  Sum15/1 -> Integrator7/1
  r-d    2/1 -> Mux1/1, Scope20/1
  "    2"/1 -> Mux10/1, Scope18/1
  Gain19/1 -> Sum36/2
  "     K 8"/1 -> Sum16/1
  Demux7/3 -> " 2"/1
  " r-d9"/1 -> Mux59/2, Scope120/1
  " r-d   10"/1 -> Mux54/3, Scope121/1
  Demux7/2 -> Mux11/2, Scope12/1
  Mux1/1 -> Scope15/1
  Demux22/2 -> Mux60/2, Scope111/1
  Mux60/1 -> Scope113/1
  Mux54/1 -> Scope114/1
  " r-d2"/1 -> Mux10/2, Scope21/1
  Mux11/1 -> Scope14/1
  Sum36/1 -> Integrator18/1
  r-d    9/1 -> Mux54/1, Scope119/1
  Demux7/7 -> " r-d2"/1
  Demux22/4 -> "    9"/1
  B2/1 -> Sum15/1
  " r-d   11"/1 -> Scope112/1
  Demux22/6 -> r-d    9/1
  Demux22/7 -> " r-d9"/1
  Mux59/1 -> Scope115/1
  Demux22/8 -> " r-d   10"/1
  "    9"/1 -> Mux59/1, Scope117/1
  "     K 4"/1 -> Sum37/1
  Sum38/1 -> "     K 4"/1
  Gain20/1 -> Sum37/2
  Uref1/1 -> Transfer Fcn5/1
  Sum17/1 -> "     K 8"/1
  Transfer Fcn5/1 -> Sum17/1
  Gain9/1 -> Sum16/2
  Integrator7/1 -> Demux7/1, Gain9/1, Gain8/1
  Demux7/4 -> "    2"/1
  " r-d   2"/1 -> Scope13/1
  Uref/1 -> Transfer Fcn2/1

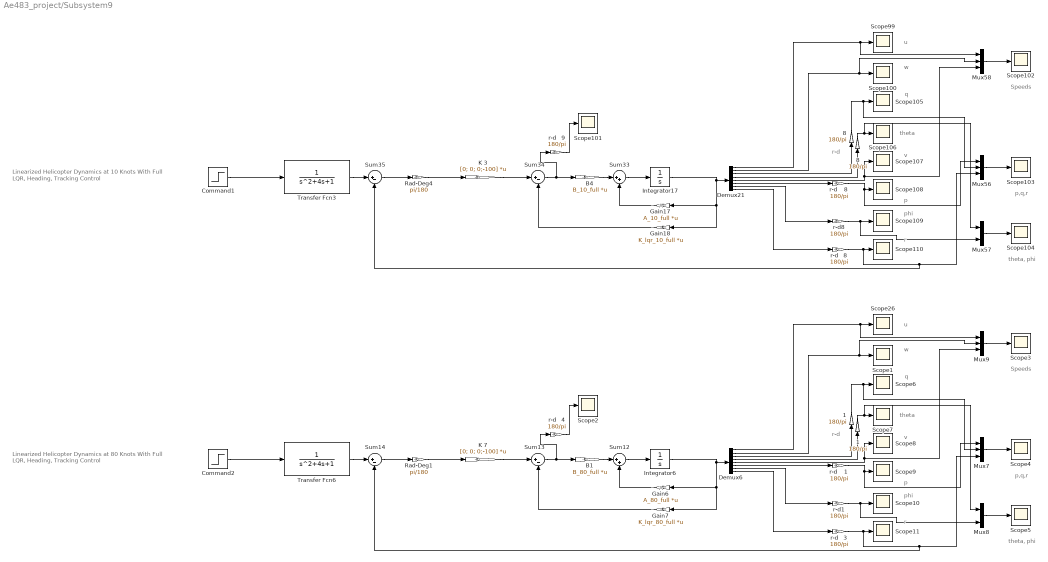
== system Ae483_project/Subsystem9 ==
  note: p
  note: phi
  note: p,q,r
  note: theta
  note: v
  note: w
  note: A
  note: r
  note: u
  note: theta, phi
  note: Speeds
  note: r-d
  note: q
  note: Linearized Helicopter
      | Dynamics at 10 Knots
      | With Full LQR, Heading, Tracking Control
  note: q
  note: Speeds
  note: theta, phi
  note: r
  note: A
  note: v
  note: p,q,r
  note: phi
  note: p
  note: Linearized Helicopter
      | Dynamics at 80 Knots
      | With Full LQR, Heading, Tracking Control
  note: u
  note: r-d
  note: w
  note: theta
  "     K 3" : Gain  Gain=[0; 0; 0;-100]  Multiplication=Matrix(K*u)
  "     K 7" : Gain  Gain=[0; 0; 0;-100]  Multiplication=Matrix(K*u)
  "    1" : Gain  Gain=180/pi
  "    8" : Gain  Gain=180/pi
  " 1" : Gain  Gain=180/pi
  " 8" : Gain  Gain=180/pi
   r-d   {3..4,8..9} (4 alike) : Gain  Gain=180/pi
  " r-d1" : Gain  Gain=180/pi
  " r-d8" : Gain  Gain=180/pi
  B1 : Gain  Gain=B_80_full  Multiplication=Matrix(K*u)
  B4 : Gain  Gain=B_10_full  Multiplication=Matrix(K*u)
  Command1 : Step  After=5  SampleTime=0
  Command2 : Step  After=5  SampleTime=0
  Demux21 : Demux  Outputs=8
  Demux6 : Demux  Outputs=8
  Gain17 : Gain  Gain=A_10_full  Multiplication=Matrix(K*u)
  Gain18 : Gain  Gain=K_lqr_10_full  Multiplication=Matrix(K*u)
  Gain6 : Gain  Gain=A_80_full  Multiplication=Matrix(K*u)
  Gain7 : Gain  Gain=K_lqr_80_full  Multiplication=Matrix(K*u)
  Integrator17 : Integrator
  Integrator6 : Integrator
  Mux{7,9,56,58} (4 alike) : Mux  Inputs=3
  Mux57 : Mux  Inputs=2
  Mux8 : Mux  Inputs=2
  Rad-Deg1 : Gain  Gain=pi/180
  Rad-Deg4 : Gain  Gain=pi/180
  Scope{1..11,26,99..110} (24 alike) : Scope
  Sum12 : Sum  Inputs=|++
  Sum{13..14,34..35} (4 alike) : Sum  Inputs=|+-
  Sum33 : Sum  Inputs=|++
  Transfer Fcn3 : TransferFcn  Denominator=[1 4 1]
  Transfer Fcn6 : TransferFcn  Denominator=[1 4 1]
  r-d    1 : Gain  Gain=180/pi
  r-d    8 : Gain  Gain=180/pi
  wires:
  Demux21/4 -> "    8"/1
  "    8"/1 -> Mux57/1, Scope106/1
  Gain7/1 -> Sum13/2
  Sum35/1 -> Rad-Deg4/1
  Gain6/1 -> Sum12/2
  Demux6/1 -> Mux9/1, Scope26/1
  " r-d   3"/1 -> Sum14/2, Mux7/3, Scope11/1
  B1/1 -> Sum12/1
  Rad-Deg4/1 -> "     K 3"/1
  Gain18/1 -> Sum34/2
  Demux21/6 -> r-d    8/1
  " 8"/1 -> Mux56/2, Scope105/1
  Demux6/8 -> " r-d   3"/1
  Sum14/1 -> Rad-Deg1/1
  " r-d1"/1 -> Mux8/2, Scope10/1
  Integrator17/1 -> Demux21/1, Gain18/1, Gain17/1
  Rad-Deg1/1 -> "     K 7"/1
  Demux21/7 -> " r-d8"/1
  " r-d8"/1 -> Mux57/2, Scope109/1
  Demux21/2 -> Mux58/2, Scope100/1
  Sum34/1 -> " r-d   9"/1, B4/1
  "     K 7"/1 -> Sum13/1
  " r-d   8"/1 -> Sum35/2, Mux56/3, Scope110/1
  Demux21/3 -> " 8"/1
  Mux57/1 -> Scope104/1
  Mux58/1 -> Scope102/1
  Demux6/2 -> Mux9/2, Scope1/1
  Transfer Fcn3/1 -> Sum35/1
  Demux6/3 -> " 1"/1
  Demux21/1 -> Mux58/1, Scope99/1
  Demux21/5 -> Mux58/3, Scope107/1
  Demux6/5 -> Mux9/3, Scope8/1
  Demux21/8 -> " r-d   8"/1
  " r-d   9"/1 -> Scope101/1
  " 1"/1 -> Mux7/2, Scope6/1
  Demux6/6 -> r-d    1/1
  Demux6/4 -> "    1"/1
  Command2/1 -> Transfer Fcn6/1
  r-d    1/1 -> Mux7/1, Scope9/1
  Sum12/1 -> Integrator6/1
  Mux7/1 -> Scope4/1
  Mux56/1 -> Scope103/1
  "     K 3"/1 -> Sum34/1
  "    1"/1 -> Mux8/1, Scope7/1
  Mux9/1 -> Scope3/1
  " r-d   4"/1 -> Scope2/1
  Command1/1 -> Transfer Fcn3/1
  Integrator6/1 -> Demux6/1, Gain7/1, Gain6/1
  B4/1 -> Sum33/1
  Gain17/1 -> Sum33/2
  Transfer Fcn6/1 -> Sum14/1
  Demux6/7 -> " r-d1"/1
  Mux8/1 -> Scope5/1
  Sum13/1 -> " r-d   4"/1, B1/1
  r-d    8/1 -> Mux56/1, Scope108/1
  Sum33/1 -> Integrator17/1

== system Ae483_project/Velocity Tracking Earth Frame ==
  note: K_w
  note: K_u
  note: K_v
  note: control rates
  note: control inputs
  note: K_angles
  note: B
  note: K
  note: transformation
      |        matrix
  note: A
  note: theta
  note: u
  note: r
  note: p,q,r
  note: w
  note: q
  note: rad-deg
  note: p
  note: phi
  note: v
  note: theta, phi,psi
  note: Speeds
  note: Linearized Helicopter
      | Dynamics at 10 Knots
      | (Model Inversion), Velocity Tracking Earth Frame
  " " : Scope
  "   " : Integrator
  "    " : Gain  Gain=B_10_full  Multiplication=Matrix(K*u)
  "     " : Gain  Gain=180/pi
  "      " : Scope
  "          " : Gain  Gain=A_10_full  Multiplication=Matrix(K*u)
  "                      " : Gain  Gain=K_10  Multiplication=Matrix(K*u)
  "                       " : Gain  Gain=[-15;15;-25]
  "                           " : Gain  Gain=L_bv_10  Multiplication=Matrix(K*u)
  "                                   " : Gain  Gain=-5  Multiplication=Matrix(K*u)
  "                                    " : Gain  Gain=[0.9;0]  Multiplication=Matrix(K*u)
  "                                     " : Derivative
  "                                         " : Scope
  "                                               " : Scope
  "                                                         " : Scope
  "                                                           " : Gain  Gain=-1  Multiplication=Matrix(K*u)
  "                                                                     " : Scope
  "                                                                                                           " : Integrator
  "                           1" : Gain  Gain=L_bv_10  Multiplication=Matrix(K*u)
  "    coeff_q" : Gain  Gain=0.000629
  "    coeff_r" : Gain  Gain=1.0024
  " 6" : Gain  Gain=180/pi
  " rad-deg       " : Gain  Gain=180/pi
  Demux10 : Demux  Outputs=3
  Demux12 : Demux  Outputs=8
  Demux13 : Demux  Outputs=3
  Mux1 : Mux  Inputs=2
  Mux{2,32..37} (7 alike) : Mux  Inputs=3
  Mux29 : Mux
  Mux31 : Mux  Inputs=2
  Scope{67..72,74..75,79} (9 alike) : Scope
  Sum{29..30,32,34..35} (5 alike) : Sum  Inputs=|+-
  Sum31 : Sum  Inputs=|++
  Sum33 : Sum  Inputs=|++
  Transfer Fcn1 : TransferFcn  Denominator=[1 4 1]
  Transfer Fcn2 : TransferFcn  Denominator=[1 4 1]
  Transfer Fcn6 : TransferFcn  Denominator=[1 4 1]
  rad-deg : Gain  Gain=180/pi
  "rad-deg  " : Gain  Gain=180/pi
  "rad-deg     " : Gain  Gain=180/pi
  "rad-deg        " : Gain  Gain=180/pi
  u_e : Step  After=20  SampleTime=0
  v_e : Step  After=5  SampleTime=0
  w_e : Step  After=10  SampleTime=0
  wires:
  Demux13/2 -> Sum30/1
  "                                                                                                           "/1 -> "rad-deg        "/1, Mux36/3
  Demux13/1 -> Sum29/1
  Demux12/6 -> Mux35/1, "rad-deg  "/1
  " rad-deg       "/1 -> Mux32/3, Scope71/1
  "                       "/1 -> Sum34/1
  Mux29/1 -> "    "/1, "rad-deg     "/1
  v_e/1 -> Mux2/2, Transfer Fcn1/1
  Sum35/1 -> "                                                           "/1
  rad-deg/1 -> Mux33/2, Scope70/1
  Demux12/7 -> rad-deg/1, Mux36/2
  Demux12/4 -> "     "/1, Mux36/1
  "rad-deg  "/1 -> Mux32/1, Scope69/1
  Sum30/1 -> "                                    "/1
  Demux12/1 -> Scope72/1, Mux34/1, Sum29/2
  Demux13/3 -> Sum35/1
  u_e/1 -> Mux2/1, Transfer Fcn6/1
  "                           "/1 -> Demux13/1
  Demux10/1 -> Mux29/1
  "                      "/1 -> Sum34/2
  Demux12/8 -> Mux35/3, "    coeff_r"/1, " rad-deg       "/1
  "   "/1 -> Demux12/1, "          "/1
  Sum29/1 -> "                                   "/1
  Transfer Fcn2/1 -> Mux37/3
  Mux33/1 -> "                                               "/1
  Transfer Fcn6/1 -> Mux37/1
  "                                    "/1 -> Mux31/2
  Demux12/3 -> "    coeff_q"/1, Mux35/2, " 6"/1
  Sum32/1 -> "                       "/1
  "     "/1 -> Mux33/1, Scope67/1
  Demux10/3 -> Mux29/4
  "    coeff_r"/1 -> Sum31/2
  w_e/1 -> Mux2/3, Transfer Fcn2/1
  Demux12/2 -> Mux34/2, Scope75/1, Sum35/2
  Mux35/1 -> "                      "/1
  Mux32/1 -> "                                                         "/1
  Mux31/1 -> Sum32/1
  "                                                           "/1 -> Mux29/2
  "          "/1 -> Sum33/2
  Mux36/1 -> Sum32/2
  Demux12/5 -> Mux34/3, Scope68/1, Sum30/2
  "    "/1 -> Sum33/1
  " 6"/1 -> Mux32/2, Scope79/1
  "rad-deg        "/1 -> Scope74/1, Mux33/3
  Demux10/2 -> Mux29/3
  Mux37/1 -> "                           "/1
  Sum31/1 -> "                                                                                                           "/1
  Sum33/1 -> "   "/1
  Sum34/1 -> Demux10/1
  "rad-deg     "/1 -> " "/1, "                                     "/1
  "                                   "/1 -> Mux31/1
  "    coeff_q"/1 -> Sum31/1
  Transfer Fcn1/1 -> Mux37/2
  "                                     "/1 -> "                                         "/1
  Mux1/1 -> "      "/1
  Mux34/1 -> Mux1/2, "                                                                     "/1
  Mux2/1 -> "                           1"/1
  "                           1"/1 -> Mux1/1
